simulink model "Events7_tmp"  (Simulink 8.3)
settings: Solver=ode45  StartTime=0.0  StopTime=10.0  RelTol=1e-3
settings Model: Creator=scaife  LastModifiedBy=bourbouh  CovSFcnEnable=on  ExtModeAutoUpdateStatusClock=off
settings DataIOCC: SignalLoggingName=sigsOut
settings OptimizationCC: InitFltsAndDblsToZero=on
settings DebuggingCC: SaveWithParameterizedLinksMsg=none  SignalResolutionControl=TryResolveAllWithWarning  SolverPrmCheckMsg=none  MultiTaskDSMMsg=warning  MultiTaskCondExecSysMsg=none  FrameProcessingCompatibilityMsg=error  StateNameClashWarn=none
settings HardwareCC: TargetUnknown=on
settings SFSimCC: SimParseCustomCode=off
settings GRTTargetCC: TargetFcnLib=ansi_tfl_tmw.mat  ModelReferenceCompliant=off  ParMdlRefBuildCompliant=off  CompOptLevelCompliant=off  ConcurrentExecutionCompliant=off  GeneratePreprocessorConditionals=Use local settings  MatFileLogging=off  MATLABClassNameForMDSCustomization=Simulink.SoftwareTarget.TargetSpecificTriggerConfigurationBase

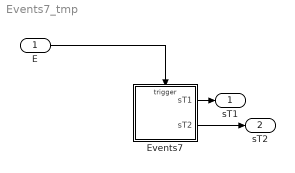
== system Events7_tmp ==
  E : Inport
  Events7 : Stateflow chart  TreatAsAtomicUnit=on
      settings: PermitHierarchicalResolution=ParametersOnly
  sT1 : Outport
  sT2 : Outport  Port=2
  wires:
  E/1 -> Events7/Trigger
  Events7/1(sT1) -> sT1/1
  Events7/2(sT2) -> sT2/1

== stateflow chart Events7 ==
  state T1 [parallel]
    settings: executionOrder=1
    state A
      en:sT1=1
    state B
      en:sT1=2
    (default) -> A
    A -> B : E
    B -> A : E
  state T2 [parallel]
    settings: executionOrder=2
    state C
      en:sT2=1
    state D
      en:sT2=2
    (default) -> C
    C -> D : enter(T1.B)
    D -> C : enter(T1.A)
  data: sT1 output double; sT2 output double
  events: E input EITHER_EDGE_EVENT
